simulink model "BoostConverterCascadedWithDC"  (R2021a)
settings: Solver=VariableStepAuto  StartTime=0.0  StopTime=10.0  RelTol=1e-3
libraries: simulink x2
settings Model: Creator=mithi  LastModifiedBy=Pallavi
settings DebuggingCC: UnconnectedInputMsg=none  UnconnectedOutputMsg=none  UnconnectedLineMsg=none
settings ModelReferenceCC: EnableRefExpFcnMdlSchedulingChecks=off
settings RTWCC: Description=Generic Real-Time Target  DLArmComputeVersion=20.02.1

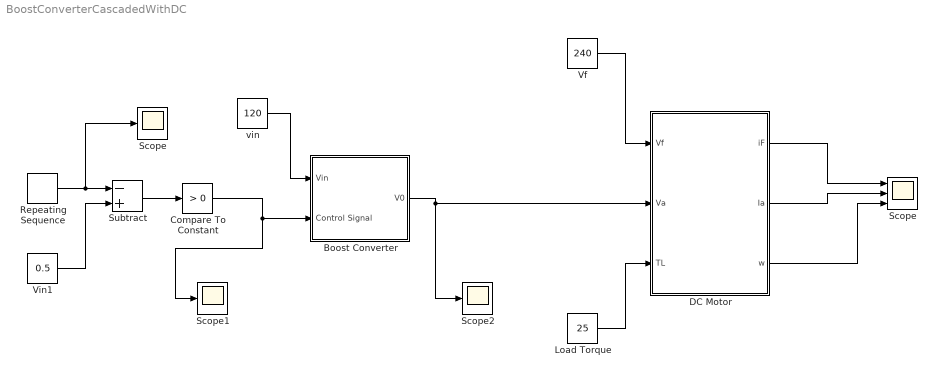
== system BoostConverterCascadedWithDC ==
  " Boost Converter" : Subsystem
  Compare To Constant : simulink/Logic and Bit Operations/Compare To Constant  relop=>  const=0  OutDataTypeStr=boolean
  DC Motor : Subsystem
  Load Torque : Constant  Value=25
  "Repeating Sequence " : simulink/Sources/Repeating Sequence  rep_seq_t=[0 2]  rep_seq_y=[0 2]
  Scope : Scope
  "Scope " : Scope  NumInputPorts=3
  Scope1 : Scope
  Scope2 : Scope
  Subtract : Sum  Inputs=-+
  Vf : Constant  Value=240
  Vin1 : Constant  Value=0.5
  vin : Constant  Value=120
  wires:
  vin/1 -> " Boost Converter"/1(Vin)
  Vin1/1 -> Subtract/2
  Compare To Constant/1 -> Scope1/1, " Boost Converter"/2(Control Signal)
  Subtract/1 -> Compare To Constant/1
  "Repeating Sequence "/1 -> Scope/1, Subtract/1
  " Boost Converter"/1(V0) -> DC Motor/2(Va), Scope2/1
  Load Torque/1 -> DC Motor/3(TL)
  Vf/1 -> DC Motor/1(Vf)
  DC Motor/1(iF) -> "Scope "/1
  DC Motor/2(Ia) -> "Scope "/2
  DC Motor/3(w) -> "Scope "/3

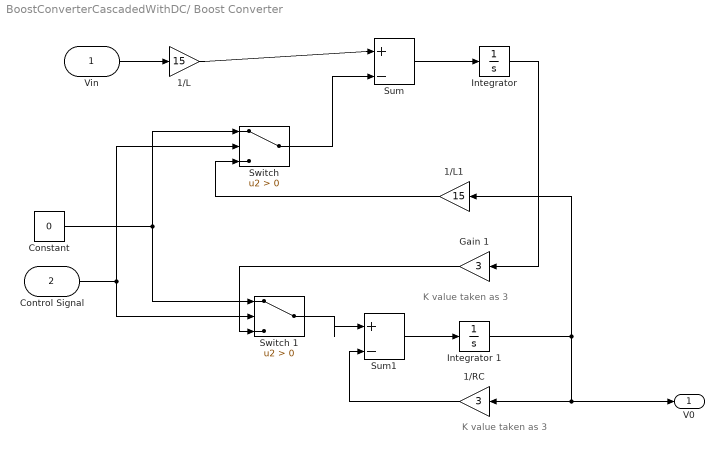
== system BoostConverterCascadedWithDC/ Boost Converter ==
  note: K value taken as 3
  note: K value taken as 3
  Vin : Inport
  Control Signal : Inport  Port=2
  1/L : Gain  Gain=15
  1/L1 : Gain  Gain=15
  1/RC : Gain  Gain=3
  "Constant " : Constant  Value=0
  Gain 1 : Gain  Gain=3
  "Integrator " : Integrator
  Integrator 1 : Integrator
  Sum : Sum  Inputs=|+-
  Sum1 : Sum  Inputs=|+-
  "Switch " : Switch  Criteria=u2 > Threshold
  Switch 1 : Switch  Criteria=u2 > Threshold
  V0 : Outport
  wires:
  "Switch "/1 -> Sum/2
  1/L/1 -> Sum/1
  Switch 1/1 -> Sum1/1
  Integrator 1/1 -> 1/RC/1, V0/1, 1/L1/1
  Sum1/1 -> Integrator 1/1
  "Constant "/1 -> Switch 1/1, "Switch "/1
  Gain 1/1 -> Switch 1/3
  "Integrator "/1 -> Gain 1/1
  Sum/1 -> "Integrator "/1
  1/L1/1 -> "Switch "/3
  Control Signal/1 -> Switch 1/2, "Switch "/2
  Vin/1 -> 1/L/1
  1/RC/1 -> Sum1/2

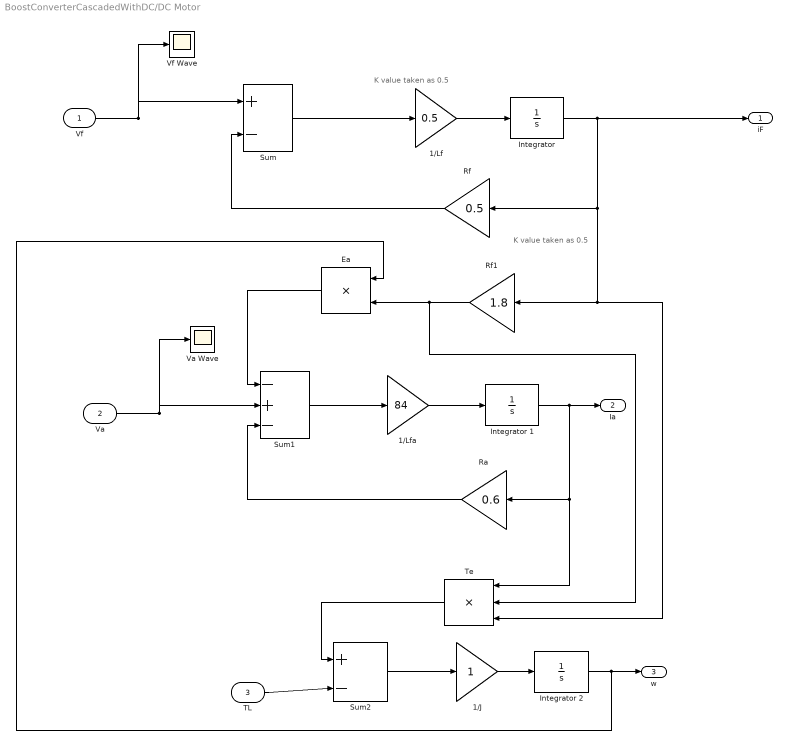
== system BoostConverterCascadedWithDC/DC Motor ==
  note: K value taken as 0.5
  note: K value taken as 0.5
  Vf : Inport
  Va : Inport  Port=2
  TL : Inport  Port=3
  1/J : Gain
  1/Lf : Gain  Gain=0.5
  1/Lfa : Gain  Gain=84
  Ea : Product
  "Integrator " : Integrator
  Integrator 1 : Integrator
  Integrator 2 : Integrator
  Ra : Gain  Gain=0.6
  Rf : Gain  Gain=0.5
  Rf1 : Gain  Gain=1.8
  Sum : Sum  Inputs=|+-
  Sum1 : Sum  Inputs=|-+-
  Sum2 : Sum  Inputs=|+-
  Te : Product  Inputs=3
  Va Wave : Scope
  Vf Wave : Scope
  iF : Outport
  Ia : Outport  Port=2
  w : Outport  Port=3
  wires:
  Sum2/1 -> 1/J/1
  Va/1 -> Sum1/2, Va Wave/1
  TL/1 -> Sum2/2
  Integrator 2/1 -> Ea/1, w/1
  Te/1 -> Sum2/1
  1/Lfa/1 -> Integrator 1/1
  Ea/1 -> Sum1/1
  Ra/1 -> Sum1/3
  "Integrator "/1 -> Rf1/1, Te/3, Rf/1, iF/1
  1/J/1 -> Integrator 2/1
  Rf1/1 -> Te/2, Ea/2
  Sum1/1 -> 1/Lfa/1
  1/Lf/1 -> "Integrator "/1
  Rf/1 -> Sum/2
  Integrator 1/1 -> Te/1, Ra/1, Ia/1
  Vf/1 -> Vf Wave/1, Sum/1
  Sum/1 -> 1/Lf/1
